simulink model "VVI_prev"  (R2022a)
settings: Solver=FixedStepAuto  StartTime=0.0  StopTime=10.0  FixedStep=1e-3  RelTol=1e-3  EnableMultiTasking=on
undefined symbols (not defined in the file): D1, D10, D11, D12, D13, D2, D3, D4, D5, D7, D8, D9, PTA0, PTA1, PTA2, PTB23, PTB9, PTC17, PTC3, PTC4, PTD0, PTD1, PTD2, PTD3
libraries: frdmk64flib x14
settings Model: ExtModeTrigDuration=5  Creator=jacqu  LastModifiedBy=yutousama
settings OptimizationCC: EnhancedBackFolding=on  PassReuseOutputArgsAs=Individual arguments  ZeroExternalMemoryAtStartup=off  ZeroInternalMemoryAtStartup=off  MaxStackSize=64  OptimizeBlockOrder=speed  DifferentSizesBufferReuse=on  OptimizationCustomize=off  EfficientTunableParamExpr=on
settings DebuggingCC: ParameterTunabilityLossMsg=error
settings HardwareCC: ProdBitPerPointer=32  ProdBitPerSizeT=32  ProdBitPerPtrDiffT=32  ProdLargestAtomicInteger=Long  ProdLargestAtomicFloat=Double  ProdWordSize=32  ProdHWDeviceType=ARM Compatible->ARM Cortex
settings SFSimCC: MATLABDynamicMemAlloc=off
settings RTWCC: SystemTargetFile=ert.tlc  HardwareBoard=NXP FRDM-K64F  TLCOptions="-aInlineSetEventsForThisBaseRateFcn=TLC_FALSE -aSuppressMultiTaskScheduler=TLC_FALSE  -aRateBasedStepFcn=0"  TemplateMakefile=ert_default_tmf  Toolchain=GNU Tools for ARM Embedded Processors
settings CodeAppCC: ForceParamTrailComments=on  IgnoreCustomStorageClasses=off  OperatorAnnotations=on  SimulinkDataObjDesc=on  SFDataObjDesc=on  InsertBlockDesc=on
settings ERTTargetCC: ExtModeTransport=4  ExtModeMexFile=sendToCommService

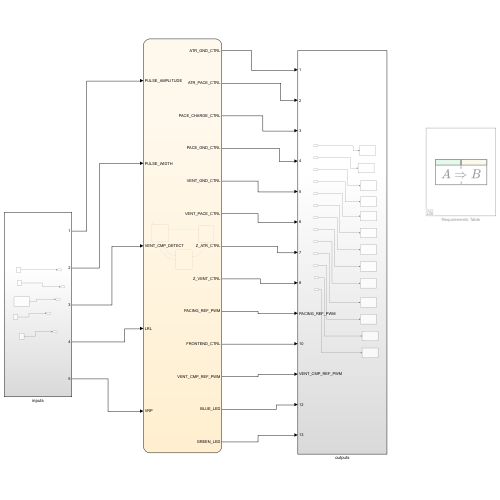
[thumbnail: Simulink's stored preview of the top-level diagram]
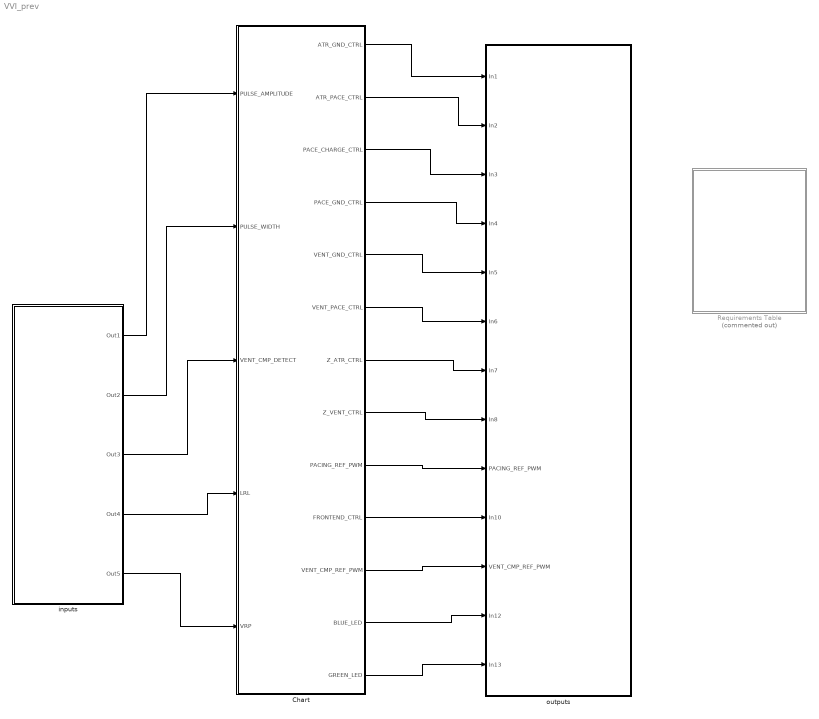
== system VVI_prev ==
  Chart : Stateflow chart  TreatAsAtomicUnit=on
  Requirements Table : Requirements Table  Commented=on  TreatAsAtomicUnit=on
  inputs : Subsystem
  outputs : Subsystem
  wires:
  inputs/1(Out1) -> Chart/1(PULSE_AMPLITUDE)
  inputs/2(Out2) -> Chart/2(PULSE_WIDTH)
  inputs/3(Out3) -> Chart/3(VENT_CMP_DETECT)
  inputs/4(Out4) -> Chart/4(LRL)
  Chart/13(GREEN_LED) -> outputs/13(In13)
  Chart/12(BLUE_LED) -> outputs/12(In12)
  Chart/11(VENT_CMP_REF_PWM) -> outputs/11(VENT_CMP_REF_PWM)
  Chart/10(FRONTEND_CTRL) -> outputs/10(In10)
  Chart/9(PACING_REF_PWM) -> outputs/9(PACING_REF_PWM)
  Chart/8(Z_VENT_CTRL) -> outputs/8(In8)
  Chart/7(Z_ATR_CTRL) -> outputs/7(In7)
  Chart/6(VENT_PACE_CTRL) -> outputs/6(In6)
  Chart/5(VENT_GND_CTRL) -> outputs/5(In5)
  Chart/3(PACE_CHARGE_CTRL) -> outputs/3(In3)
  Chart/4(PACE_GND_CTRL) -> outputs/4(In4)
  Chart/2(ATR_PACE_CTRL) -> outputs/2(In2)
  Chart/1(ATR_GND_CTRL) -> outputs/1(In1)
  inputs/5(Out5) -> Chart/5(VRP)

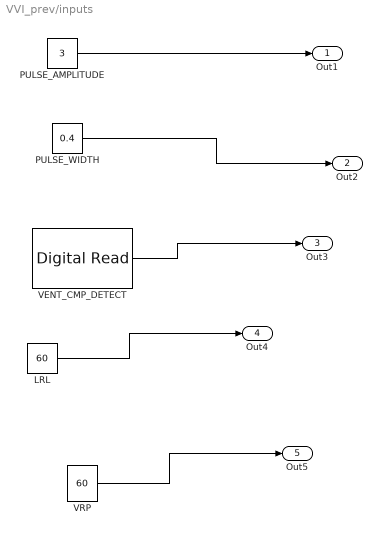
== system VVI_prev/inputs ==
  LRL : Constant  Value=60
  PULSE_AMPLITUDE : Constant  Value=3
  PULSE_WIDTH : Constant  Value=0.4
  VENT_CMP_DETECT : frdmk64flib/Digital Read  Whichpin=PTC17 (D1)  SampleTime=-1
  VRP : Constant  Value=60
  Out1 : Outport
  Out2 : Outport  Port=2
  Out3 : Outport  Port=3
  Out4 : Outport  Port=4
  Out5 : Outport  Port=5
  wires:
  PULSE_AMPLITUDE/1 -> Out1/1
  VENT_CMP_DETECT/1 -> Out3/1
  LRL/1 -> Out4/1
  PULSE_WIDTH/1 -> Out2/1
  VRP/1 -> Out5/1

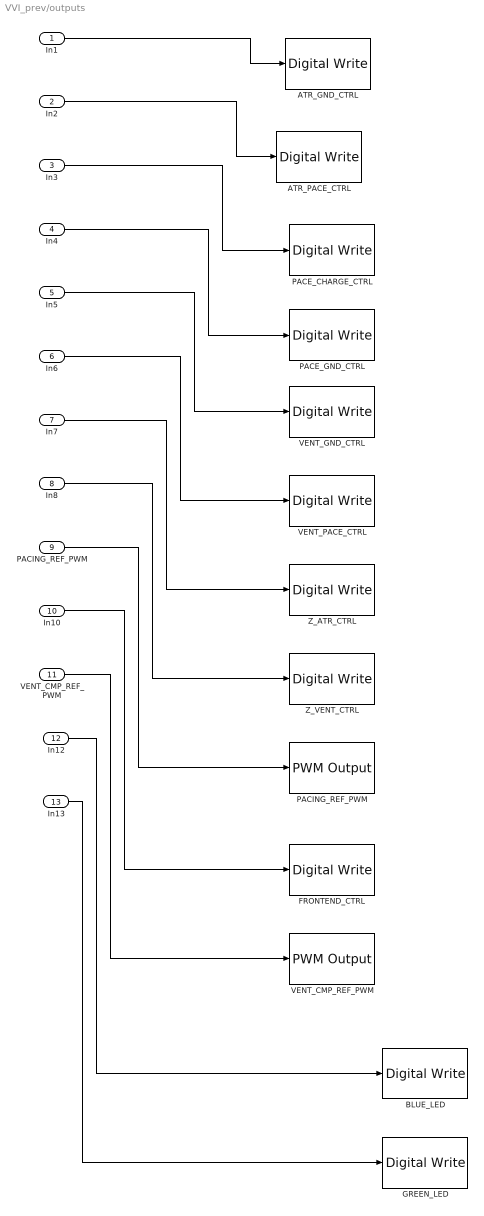
== system VVI_prev/outputs ==
  In1 : Inport
  In2 : Inport  Port=2
  In3 : Inport  Port=3
  In4 : Inport  Port=4
  In5 : Inport  Port=5
  In6 : Inport  Port=6
  In7 : Inport  Port=7
  In8 : Inport  Port=8
  PACING_REF_PWM : Inport  Port=9
  In10 : Inport  Port=10
  VENT_CMP_REF_PWM : Inport  Port=11
  In12 : Inport  Port=12
  In13 : Inport  Port=13
  " PACING_REF_PWM" : frdmk64flib/PWM Output  Whichpin=PTA2 (D5)  InitialFrequency=2000  InitialDutyCycle=0
  " VENT_CMP_REF_PWM" : frdmk64flib/PWM Output  Whichpin=PTA1 (D3)  InitialFrequency=2000  InitialDutyCycle=0
  ATR_GND_CTRL : frdmk64flib/Digital Write  Whichpin=PTD2 (D11)
  ATR_PACE_CTRL : frdmk64flib/Digital Write  Whichpin=PTA0 (D8)
  BLUE_LED : frdmk64flib/Digital Write  Whichpin=BLUE_LED
  FRONTEND_CTRL : frdmk64flib/Digital Write  Whichpin=PTD1 (D13)
  GREEN_LED : frdmk64flib/Digital Write  Whichpin=GREEN_LED
  PACE_CHARGE_CTRL : frdmk64flib/Digital Write  Whichpin=PTB9 (D2)
  PACE_GND_CTRL : frdmk64flib/Digital Write  Whichpin=PTD0 (D10)
  VENT_GND_CTRL : frdmk64flib/Digital Write  Whichpin=PTD3 (D12)
  VENT_PACE_CTRL : frdmk64flib/Digital Write  Whichpin=PTC4 (D9)
  Z_ATR_CTRL : frdmk64flib/Digital Write  Whichpin=PTB23 (D4)
  Z_VENT_CTRL : frdmk64flib/Digital Write  Whichpin=PTC3 (D7)
  wires:
  In10/1 -> FRONTEND_CTRL/1
  In12/1 -> BLUE_LED/1
  In13/1 -> GREEN_LED/1
  VENT_CMP_REF_PWM/1 -> " VENT_CMP_REF_PWM"/1
  In7/1 -> Z_ATR_CTRL/1
  In3/1 -> PACE_CHARGE_CTRL/1
  In2/1 -> ATR_PACE_CTRL/1
  In1/1 -> ATR_GND_CTRL/1
  In8/1 -> Z_VENT_CTRL/1
  In5/1 -> VENT_GND_CTRL/1
  PACING_REF_PWM/1 -> " PACING_REF_PWM"/1
  In6/1 -> VENT_PACE_CTRL/1
  In4/1 -> PACE_GND_CTRL/1

== stateflow chart VVI_prev/Requirements Table ==
  (default) -> (junction 1073748787)
  (junction 1073748787) -> (junction 1073748788) : {
      | % SF_REQ_REV_07
      | }
  (junction 1073748788) -> (junction 1073748790) : {
      | % HEADER_ASSIGNMENTS
      |
      | }
  (junction 1073748790) -> (junction 1073748792) : {
      | % START_A_4
      | }
  (junction 1073748792) -> (junction 1073748794) : {
      | }
  (junction 1073748794) -> (junction 1073748796)
  (junction 1073748796) -> (junction 1073748798) : {
      | }
  (junction 1073748798) -> (junction 1073748800) : {
      | % END_A_4
      | }
  (junction 1073748800) -> (junction 1073748802) : {
      | % START_R_1
      | }
  (junction 1073748802) -> (junction 1073748804) : {
      | }
  (junction 1073748804) -> (junction 1073748806) : {
      |
      |
      | }
  (junction 1073748806) -> (junction 1073748808) : {
      | }
  (junction 1073748808) -> (junction 1073748810) : {
      | % START_R_7
      | }
  (junction 1073748810) -> (junction 1073748812) : {
      | }
  (junction 1073748812) -> (junction 1073748814)
  (junction 1073748814) -> (junction 1073748816) [order 1] : [(prev(FRONTEND_CTRL)==true) && (prev(PACE_CHARGE_CTRL)==true) && (prev(VENT_PACE_CTRL)==false) && (prev(VENT_GND_CTRL)==false) && (prev(BLUE_LED)==false) && (prev(GREEN_LED)==false) && (prev(ATR_GND_CTRL)==true)]
  (junction 1073748814) -> (junction 1073748858) [order 2]
  (junction 1073748816) -> (junction 1073748818) : {
      |
      |
      | }
  (junction 1073748818) -> (junction 1073748820) : {
      | }
  (junction 1073748820) -> (junction 1073748822) : {
      | % START_R_16
      | }
  (junction 1073748822) -> (junction 1073748824) : {
      | }
  (junction 1073748824) -> (junction 1073748826)
  (junction 1073748826) -> (junction 1073748828) [order 1] : [duration((prev(VENT_CMP_DETECT)==false)) >= ((60000/HEART_RATE)-PULSE_WIDTH)/1000]
  (junction 1073748826) -> (junction 1073748834) [order 2]
  (junction 1073748828) -> (junction 1073748830) : {
      | reqtable_postcondition((VENT_PACE_CTRL==true) && (PACE_CHARGE_CTRL==false) && (VENT_PACE_CTRL==true) && (VENT_GND_CTRL==false) && (FRONTEND_CTRL==true) && (BLUE_LED==true) && (ATR_GND_CTRL==false), 'R:1.1.1');
      |
      |
      | }
  (junction 1073748830) -> (junction 1073748832) : {
      | }
  (junction 1073748832) -> (junction 1073748834)
  (junction 1073748834) -> (junction 1073748836)
  (junction 1073748836) -> (junction 1073748838) : {
      | % END_R_16
      | }
  (junction 1073748838) -> (junction 1073748840) : {
      | % START_R_22
      | }
  (junction 1073748840) -> (junction 1073748842) : {
      | }
  (junction 1073748842) -> (junction 1073748844)
  (junction 1073748844) -> (junction 1073748846) [order 1] : [(prev(VENT_CMP_DETECT)==true)]
  (junction 1073748844) -> (junction 1073748852) [order 2]
  (junction 1073748846) -> (junction 1073748848) : {
      | reqtable_postcondition((VENT_PACE_CTRL==false) && (PACE_CHARGE_CTRL==false) && (VENT_PACE_CTRL==false) && (VENT_GND_CTRL==true) && (FRONTEND_CTRL==false) && (GREEN_LED==true), 'R:1.1.2');
      |
      |
      | }
  (junction 1073748848) -> (junction 1073748850) : {
      | }
  (junction 1073748850) -> (junction 1073748852)
  (junction 1073748852) -> (junction 1073748854)
  (junction 1073748854) -> (junction 1073748856) : {
      | % END_R_22
      | }
  (junction 1073748856) -> (junction 1073748858)
  (junction 1073748858) -> (junction 1073748860)
  (junction 1073748860) -> (junction 1073748862) : {
      | % END_R_7
      | }
  (junction 1073748862) -> (junction 1073748864) : {
      | % START_R_10
      | }
  (junction 1073748864) -> (junction 1073748866) : {
      | }
  (junction 1073748866) -> (junction 1073748868)
  (junction 1073748868) -> (junction 1073748870) [order 1] : [(prev(FRONTEND_CTRL)==true) && (prev(PACE_CHARGE_CTRL)==false) && (prev(VENT_PACE_CTRL)==true) && (prev(VENT_GND_CTRL)==false) && (prev(BLUE_LED)==true) && (prev(GREEN_LED)==false) && (prev(ATR_GND_CTRL)==false)]
  (junction 1073748868) -> (junction 1073748912) [order 2]
  (junction 1073748870) -> (junction 1073748872) : {
      |
      |
      | }
  (junction 1073748872) -> (junction 1073748874) : {
      | }
  (junction 1073748874) -> (junction 1073748876) : {
      | % START_R_25
      | }
  (junction 1073748876) -> (junction 1073748878) : {
      | }
  (junction 1073748878) -> (junction 1073748880)
  (junction 1073748880) -> (junction 1073748882) [order 1] : [duration((prev(VENT_CMP_DETECT)==false)) >= PULSE_WIDTH/1000]
  (junction 1073748880) -> (junction 1073748888) [order 2]
  (junction 1073748882) -> (junction 1073748884) : {
      | reqtable_postcondition((VENT_PACE_CTRL==false) && (PACE_CHARGE_CTRL==true) && (VENT_PACE_CTRL==false) && (VENT_GND_CTRL==false) && (FRONTEND_CTRL==true) && (BLUE_LED==false) && (ATR_GND_CTRL==true), 'R:1.2.1');
      |
      |
      | }
  (junction 1073748884) -> (junction 1073748886) : {
      | }
  (junction 1073748886) -> (junction 1073748888)
  (junction 1073748888) -> (junction 1073748890)
  (junction 1073748890) -> (junction 1073748892) : {
      | % END_R_25
      | }
  (junction 1073748892) -> (junction 1073748894) : {
      | % START_R_28
      | }
  (junction 1073748894) -> (junction 1073748896) : {
      | }
  (junction 1073748896) -> (junction 1073748898)
  (junction 1073748898) -> (junction 1073748900) [order 1] : [(prev(VENT_CMP_DETECT)==true)]
  (junction 1073748898) -> (junction 1073748906) [order 2]
  (junction 1073748900) -> (junction 1073748902) : {
      | reqtable_postcondition((VENT_PACE_CTRL==false) && (PACE_CHARGE_CTRL==false) && (VENT_PACE_CTRL==false) && (VENT_GND_CTRL==true) && (FRONTEND_CTRL==false) && (GREEN_LED==true), 'R:1.2.2');
      |
      |
      | }
  (junction 1073748902) -> (junction 1073748904) : {
      | }
  (junction 1073748904) -> (junction 1073748906)
  (junction 1073748906) -> (junction 1073748908)
  (junction 1073748908) -> (junction 1073748910) : {
      | % END_R_28
      | }
  (junction 1073748910) -> (junction 1073748912)
  (junction 1073748912) -> (junction 1073748914)
  (junction 1073748914) -> (junction 1073748916) : {
      | % END_R_10
      | }
  (junction 1073748916) -> (junction 1073748918) : {
      | % START_R_13
      | }
  (junction 1073748918) -> (junction 1073748920) : {
      | }
  (junction 1073748920) -> (junction 1073748922)
  (junction 1073748922) -> (junction 1073748924) [order 1] : [(prev(FRONTEND_CTRL)==false) && (prev(PACE_CHARGE_CTRL)==false) && (prev(VENT_PACE_CTRL)==false) && (prev(VENT_GND_CTRL)==true)]
  (junction 1073748922) -> (junction 1073748930) [order 2]
  (junction 1073748924) -> (junction 1073748926) : {
      | reqtable_postcondition((BLUE_LED==false) && (PACE_CHARGE_CTRL==true) && (VENT_PACE_CTRL==false) && (VENT_GND_CTRL==false) && (FRONTEND_CTRL==true) && (GREEN_LED==false) && (ATR_GND_CTRL==true), 'R:1.3');
      |
      |
      | }
  (junction 1073748926) -> (junction 1073748928) : {
      | }
  (junction 1073748928) -> (junction 1073748930)
  (junction 1073748930) -> (junction 1073748932)
  (junction 1073748932) -> (junction 1073748934) : {
      | % END_R_13
      | }
  (junction 1073748934) -> (junction 1073748936) : {
      | % END_R_1
      | }

== stateflow chart VVI_prev/Chart ==
  note: when vent_cmp_detect = 0, paceon mode.
  state PACE_OFF
    entry:
    ATR_PACE_CTRL = 0
    VENT_PACE_CTRL = 0
    PACING_REF_PWM = 20*PULSE_AMPLITUDE
    PACE_CHARGE_CTRL = 1
    PACE_GND_CTRL = 1
    VENT_PACE_CTRL = 0
    Z_ATR_CTRL = 0
    Z_VENT_CTRL = 0
    ATR_PACE_CTRL = 0
    ATR_GND_CTRL = 1
    VENT_GND_CTRL = 0
    FRONTEND_CTRL = 1
    VENT_CMP_REF_PWM = 20*PULSE_AMPLITUDE
    % light indicators
    BLUE_LED = 0
    GREEN_LED = 0
  state PACE_ON
    entry:
    PACE_CHARGE_CTRL = 0
    PACE_GND_CTRL = 1
    ATR_PACE_CTRL = 0
    ATR_GND_CTRL = 0
    Z_ATR_CTRL = 0
    Z_VENT_CTRL = 0
    VENT_GND_CTRL = 0
    VENT_PACE_CTRL = 1
    % light indicator
    BLUE_LED = 1
  note: at pace_off state and wait for the vent_cmp_detect signal to decide which
      | mode to go to.
  note: vent_cmp_detect = 1, the heart works fine, so refractory mode
  state REFRACTORY
    entry:
    FRONTEND_CTRL = 0
    VENT_PACE_CTRL = 0
    VENT_GND_CTRL = 1
    PACING_REF_PWM = 20*PULSE_AMPLITUDE
    PACE_CHARGE_CTRL = 0
    PACE_GND_CTRL = 1
    % light indicator
    GREEN_LED = 1
  (default) -> PACE_OFF
  PACE_OFF -> PACE_ON [order 1] : [(VENT_CMP_DETECT == 0) & after((60000/LRL)-PULSE_WIDTH-VRP,msec)]
  PACE_ON -> REFRACTORY : [after(PULSE_WIDTH,msec)]
  REFRACTORY -> PACE_OFF : [after(VRP,msec)]
  PACE_OFF -> REFRACTORY [order 2] : [VENT_CMP_DETECT == 1]
  data: ATR_GND_CTRL output; ATR_PACE_CTRL output; PACE_CHARGE_CTRL output; PACE_GND_CTRL output; VENT_GND_CTRL output; VENT_PACE_CTRL output; Z_ATR_CTRL output; Z_VENT_CTRL output; PULSE_AMPLITUDE input; PACING_REF_PWM output; FRONTEND_CTRL output; VENT_CMP_REF_PWM output; BLUE_LED output; PULSE_WIDTH input; VENT_CMP_DETECT input; GREEN_LED output; LRL input; VRP input
